simulink model "electrical_reduced_order_to_pdf"  (R2015b)
settings: Solver=VariableStepAuto  StartTime=0.0  StopTime=10.0  RelTol=1e-3
undefined symbols (not defined in the file): J, Kt, Kv, R, Vin
settings Model: Creator=Morten  LastModifiedBy=Morten

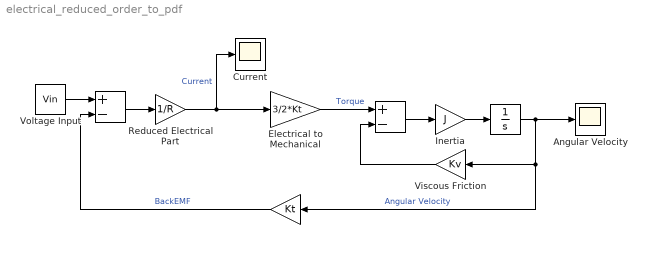
== system electrical_reduced_order_to_pdf ==
  "  " : Sum  Inputs=+-
  "      " : Sum  Inputs=+-
  "                            " : Gain  Gain=Kt
  "                                     " : Integrator
  Angular Velocity : Scope
  Current : Scope
  Electrical to Mechanical : Gain  Gain=3/2*Kt
  Inertia : Gain  Gain=J
  Reduced Electrical Part : Gain  Gain=1/R
  Viscous Friction : Gain  Gain=Kv
  Voltage Input : Constant  Value=Vin
  wires:
  "      "/1 -> Inertia/1
  Reduced Electrical Part/1 -> Current/1, Electrical to Mechanical/1  "Current"
  "                            "/1 -> "  "/2  "BackEMF"
  Inertia/1 -> "                                     "/1
  "  "/1 -> Reduced Electrical Part/1
  Voltage Input/1 -> "  "/1
  "                                     "/1 -> Angular Velocity/1, "                            "/1, Viscous Friction/1  "Angular Velocity"
  Electrical to Mechanical/1 -> "      "/1  "Torque"
  Viscous Friction/1 -> "      "/2
